simulink model "RIP"  (Simulink 8.9)
settings: Solver=ode45  StartTime=0.0  StopTime=30  RelTol=1e-6  EnableMultiTasking=on
undefined symbols (not defined in the file): d0, d1, g, J0, J1, Kf, Kg, Kt, L0, L1, m1, Ra
settings Model: Creator=Alvin  LastModifiedBy=Alvin
settings SolverCC: AlgebraicLoopSolver=LineSearch
settings DataIOCC: SignalLoggingSaveFormat=Dataset  SaveState=on
settings DebuggingCC: UnderspecifiedInitializationDetection=Simplified  MergeDetectMultiDrivingBlocksExec=error  FcnCallInpInsideContextMsg=error  StateNameClashWarn=none
settings GRTTargetCC: CombineOutputUpdateFcns=on  GRTInterface=off

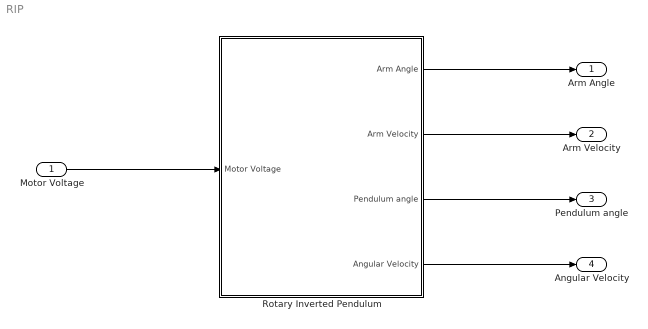
== system RIP ==
  Motor Voltage : Inport
  Rotary Inverted Pendulum : Subsystem
  Arm Angle : Outport
  Arm Velocity : Outport  Port=2
  Pendulum angle : Outport  Port=3
  Angular Velocity : Outport  Port=4
  wires:
  Motor Voltage/1 -> Rotary Inverted Pendulum/1(Motor Voltage)
  Rotary Inverted Pendulum/1(Arm Angle) -> Arm Angle/1
  Rotary Inverted Pendulum/2(Arm Velocity) -> Arm Velocity/1
  Rotary Inverted Pendulum/3(Pendulum angle) -> Pendulum angle/1
  Rotary Inverted Pendulum/4(Angular Velocity) -> Angular Velocity/1

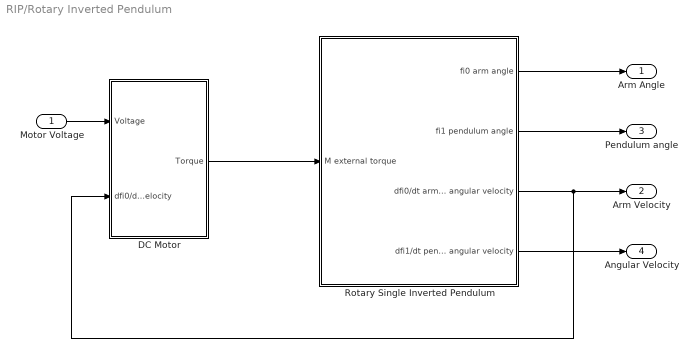
== system RIP/Rotary Inverted Pendulum ==
  Motor Voltage : Inport
  DC Motor : Subsystem
  Rotary Single Inverted Pendulum : Subsystem
  Arm Angle : Outport
  Arm Velocity : Outport  Port=2
  Pendulum angle : Outport  Port=3
  Angular Velocity : Outport  Port=4
  wires:
  Rotary Single Inverted Pendulum/2(fi1 pendulum angle) -> Pendulum angle/1
  Rotary Single Inverted Pendulum/4(dfi1/dt pendulum angular velocity) -> Angular Velocity/1
  Motor Voltage/1 -> DC Motor/1(Voltage)
  Rotary Single Inverted Pendulum/3(dfi0/dt arm angular velocity) -> Arm Velocity/1, DC Motor/2(dfi0/dt Arm Angular Velocity)
  DC Motor/1(Torque) -> Rotary Single Inverted Pendulum/1(M external torque)
  Rotary Single Inverted Pendulum/1(fi0 arm angle) -> Arm Angle/1

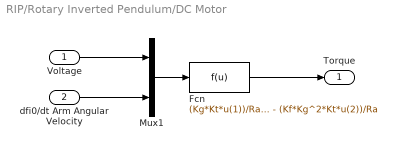
== system RIP/Rotary Inverted Pendulum/DC Motor ==
  Voltage : Inport
  dfi0/dt Arm Angular Velocity : Inport  Port=2
  Fcn : Fcn  Expr=(Kg*Kt*u(1))/Ra - (Kf*Kg^2*Kt*u(2))/Ra
  Mux1 : Mux  Inputs=2
  Torque : Outport
  wires:
  dfi0/dt Arm Angular Velocity/1 -> Mux1/2
  Voltage/1 -> Mux1/1
  Mux1/1 -> Fcn/1
  Fcn/1 -> Torque/1

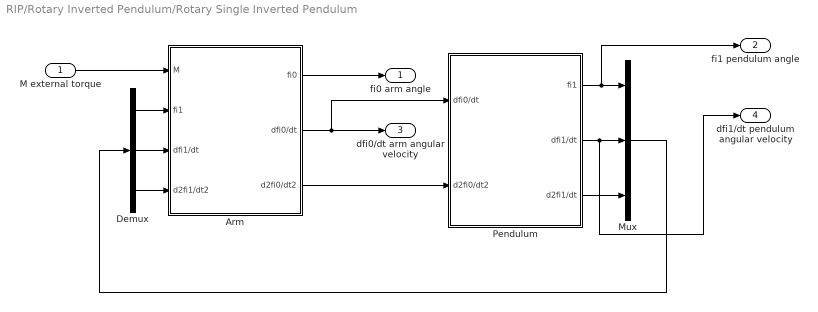
== system RIP/Rotary Inverted Pendulum/Rotary Single Inverted Pendulum ==
  M external torque : Inport
  Arm : Subsystem
  Demux : Demux  Outputs=3
  Mux : Mux  Inputs=3
  Pendulum : Subsystem
  fi0 arm angle : Outport
  fi1 pendulum angle : Outport  Port=2
  dfi0/dt arm angular velocity : Outport  Port=3
  dfi1/dt pendulum angular velocity : Outport  Port=4
  wires:
  Pendulum/1(fi1) -> fi1 pendulum angle/1, Mux/1
  Pendulum/2(dfi1/dt) -> dfi1/dt pendulum angular velocity/1, Mux/2
  Mux/1 -> Demux/1
  Demux/1 -> Arm/2(fi1)
  Demux/2 -> Arm/3(dfi1/dt)
  Demux/3 -> Arm/4(d2fi1/dt2)
  M external torque/1 -> Arm/1(M)
  Pendulum/3(d2fi1/dt) -> Mux/3
  Arm/3(d2fi0/dt2) -> Pendulum/2(d2fi0/dt2)
  Arm/1(fi0) -> fi0 arm angle/1
  Arm/2(dfi0/dt) -> dfi0/dt arm angular velocity/1, Pendulum/1(dfi0/dt)

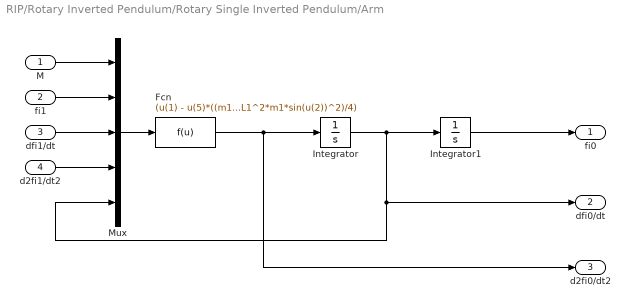
== system RIP/Rotary Inverted Pendulum/Rotary Single Inverted Pendulum/Arm ==
  M : Inport
  fi1 : Inport  Port=2
  dfi1/dt : Inport  Port=3
  d2fi1/dt2 : Inport  Port=4
  Fcn : Fcn  Expr=(u(1) - u(5)*((m1*u(3)*sin(2*u(2))*L1^2)/4 + d0) + (L0*L1*m1*u(3)^2*sin(u(2)))/2 - (L0*L1*m1*u(4)*cos(u(2)))/2)/(J0 + L0^2*m1 + (L1^2*m1*sin(u(2))^2)/4)
  Integrator : Integrator
  Integrator1 : Integrator
  Mux : Mux  Inputs=5
  fi0 : Outport
  dfi0/dt : Outport  Port=2
  d2fi0/dt2 : Outport  Port=3
  wires:
  Mux/1 -> Fcn/1
  Fcn/1 -> d2fi0/dt2/1, Integrator/1
  Integrator/1 -> dfi0/dt/1, Mux/5, Integrator1/1
  Integrator1/1 -> fi0/1
  fi1/1 -> Mux/2
  dfi1/dt/1 -> Mux/3
  M/1 -> Mux/1
  d2fi1/dt2/1 -> Mux/4

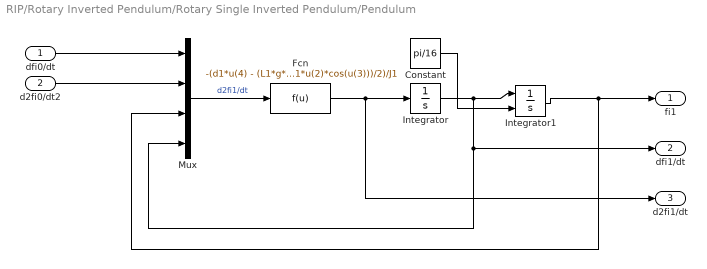
== system RIP/Rotary Inverted Pendulum/Rotary Single Inverted Pendulum/Pendulum ==
  dfi0/dt : Inport
  d2fi0/dt2 : Inport  Port=2
  Constant : Constant  Value=pi/16
  Fcn : Fcn  Expr=-(d1*u(4) - (L1*g*m1*sin(u(3)))/2 - (L1^2*m1*u(1)^2*sin(2*u(3)))/8 + (L0*L1*m1*u(2)*cos(u(3)))/2)/J1
  Integrator : Integrator
  Integrator1 : Integrator  InitialConditionSource=external
  Mux : Mux
  fi1 : Outport
  dfi1/dt : Outport  Port=2
  d2fi1/dt : Outport  Port=3
  wires:
  Integrator1/1 -> fi1/1, Mux/3
  Fcn/1 -> d2fi1/dt/1, Integrator/1
  Mux/1 -> Fcn/1  "d2fi1/dt"
  Integrator/1 -> dfi1/dt/1, Mux/4, Integrator1/1
  dfi0/dt/1 -> Mux/1
  d2fi0/dt2/1 -> Mux/2
  Constant/1 -> Integrator1/2
